simulink model "DC_DC_source_based_matrix_switches1_2022a"  (R2023a)
settings: Solver=FixedStepAuto  StartTime=0.0  StopTime=10000  RelTol=1e-3
InitFcn:
  | %run('D:\Thesis\main.m')
  | %run('E:\Thesis\main.m')
values from neighbouring files (symbols this model uses):
  cell_cap_Ah = 2.2    [find_maximum_ovlp.m]    (also in main.m)
  dst_q_cls = zeros(50, 2)    [main.m]
  dst_trg_soc_av = zeros(50, 1)    [main.m]
  soc = soc_in    [balance_costF.m]    (also in find_maximum_ovlp.m = fix(rand (1, cell_count) * 100); log_clustering.m; main.m = fix(rand (1, cell_count) * 100); plot_final.m)
  src_q_cls = zeros(50, 2)    [main.m]
  src_trg_soc_av = zeros(50, 1)    [main.m]
undefined symbols (not defined in the file or in its folder): Ion, Lithium
libraries: spsIdealSwitchLib x18, spsBatteryLib x9, spsControlledCurrentSourceLib x2, spsVoltageMeasurementLib x2, spsOnDelayLib x1, spsSeriesRLCBranchLib x1, spspowerguiLib x1
settings Model: Creator=Mahdi  LastModifiedBy=10661025
settings OptimizationCC: DefaultParameterBehavior=Inlined  EnhancedBackFolding=on  PassReuseOutputArgsAs=Individual arguments  ZeroExternalMemoryAtStartup=off  ZeroInternalMemoryAtStartup=off  OptimizeBlockOrder=speed  DifferentSizesBufferReuse=on  OptimizationCustomize=off  EfficientTunableParamExpr=on
settings DebuggingCC: ParameterTunabilityLossMsg=error
settings HardwareCC: ProdBitPerInt=16  ProdBitPerPointer=16  ProdBitPerSizeT=16  ProdBitPerPtrDiffT=16  ProdLargestAtomicFloat=None  ProdWordSize=16  ProdHWDeviceType=STMicroelectronics->ST10/Super10
settings ModelReferenceCC: ModelReferenceMinAlgLoopOccurrences=on
settings SFSimCC: MATLABDynamicMemAlloc=off
settings RTWCC: Description=Embedded Coder  SystemTargetFile=ert.tlc  TemplateMakefile=ert_default_tmf
settings CodeAppCC: ForceParamTrailComments=on  IgnoreCustomStorageClasses=off  OperatorAnnotations=on  SimulinkDataObjDesc=on  SFDataObjDesc=on  InsertBlockDesc=on
settings ERTTargetCC: TargetLangStandard=C99 (ISO)  GenerateSampleERTMain=on  SupportContinuousTime=on  SupportVariableSizeSignals=on  InlinedParameterPlacement=NonHierarchical  ERTCustomFileTemplate=example_file_process.tlc

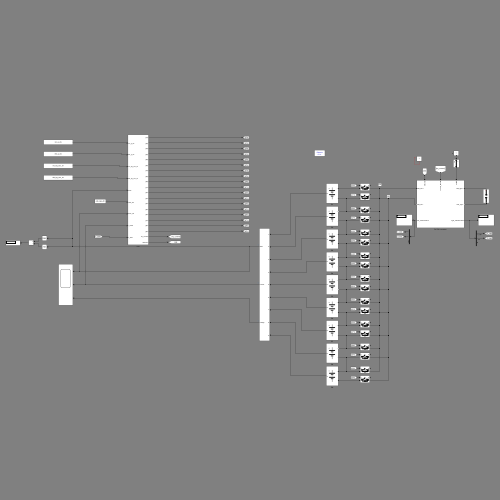
[thumbnail: Simulink's stored preview of the top-level diagram]
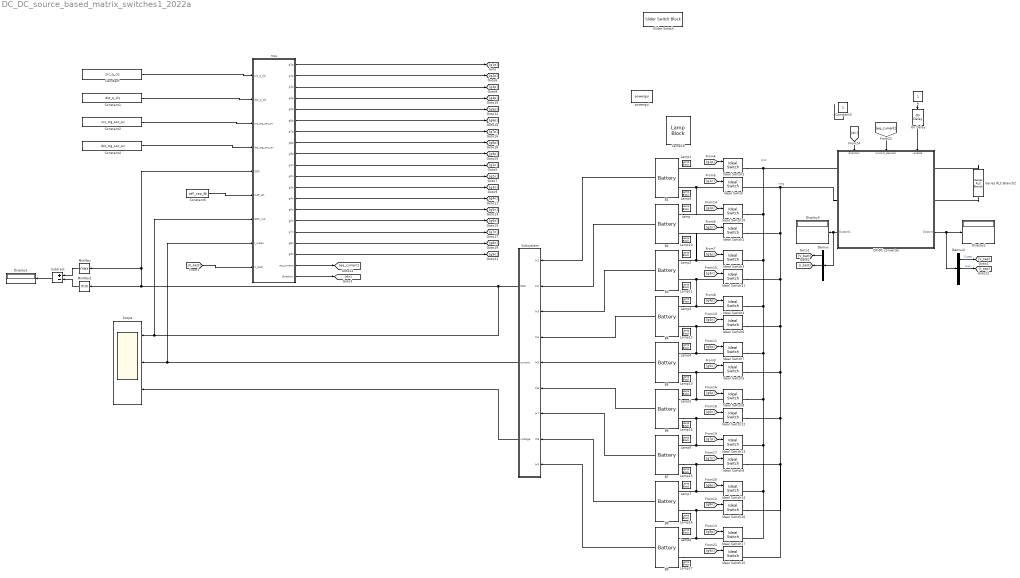
== system DC_DC_source_based_matrix_switches1_2022a ==
  note: pos
  note: neg
  B1 : spsBatteryLib/Battery  BatType=Lithium-Ion  ShowTempParam=off  ThermalPreset=no  ShowAgeParam=off  NomV=3.7  NomQ=2.2  SOC=soc(1, 1)  Batt_Tr=30  PresetModel=on  MaxQ=2.2  MinV=2.775  FullV=4.3068  Dis_rate=0.95652  R=0.016818  Normal_OP=1.9896  expZone="[3.9974     0.10809]"  current=[6.5 13 32.5]  Units=Time  Tci=20  NomT=20  T2=-30  MaxQ2=4.8  FullV2=7.1  Normal_OP2=5.655  expZone2="[6.58           1]"  Rca=0.6  ti=2000  Dp=0  Neq0=0  Tsim=1e6  Ta1=25  Qeol=5.4*0.9  Reol=0.013333*1.2  Char_age=[2.3478, 3]  Dis_age=[2.3478, 10]  N1=1500  N2=10500  N3=1000  N4=1400  Ta2=45  N5=950
  B2 : spsBatteryLib/Battery  BatType=Lithium-Ion  ShowTempParam=off  ThermalPreset=no  ShowAgeParam=off  NomV=3.7  NomQ=2.2  SOC=soc(1, 2)  Batt_Tr=30  PresetModel=on  MaxQ=2.2  MinV=2.775  FullV=4.3068  Dis_rate=0.95652  R=0.016818  Normal_OP=1.9896  expZone="[3.9974     0.10809]"  current=[6.5 13 32.5]  Units=Time  Tci=20  NomT=20  T2=-30  MaxQ2=4.8  FullV2=7.1  Normal_OP2=5.655  expZone2="[6.58           1]"  Rca=0.6  ti=2000  Dp=0  Neq0=0  Tsim=1e6  Ta1=25  Qeol=5.4*0.9  Reol=0.013333*1.2  Char_age=[2.3478, 3]  Dis_age=[2.3478, 10]  N1=1500  N2=10500  N3=1000  N4=1400  Ta2=45  N5=950
  B3 : spsBatteryLib/Battery  BatType=Lithium-Ion  ShowTempParam=off  ThermalPreset=no  ShowAgeParam=off  NomV=3.7  NomQ=2.2  SOC=soc(1, 3)  Batt_Tr=30  PresetModel=on  MaxQ=2.2  MinV=2.775  FullV=4.3068  Dis_rate=0.95652  R=0.016818  Normal_OP=1.9896  expZone="[3.9974     0.10809]"  current=[6.5 13 32.5]  Units=Time  Tci=20  NomT=20  T2=-30  MaxQ2=4.8  FullV2=7.1  Normal_OP2=5.655  expZone2="[6.58           1]"  Rca=0.6  ti=2000  Dp=0  Neq0=0  Tsim=1e6  Ta1=25  Qeol=5.4*0.9  Reol=0.013333*1.2  Char_age=[2.3478, 3]  Dis_age=[2.3478, 10]  N1=1500  N2=10500  N3=1000  N4=1400  Ta2=45  N5=950
  B4 : spsBatteryLib/Battery  BatType=Lithium-Ion  ShowTempParam=off  ThermalPreset=no  ShowAgeParam=off  NomV=3.7  NomQ=2.2  SOC=soc(1, 4)  Batt_Tr=30  PresetModel=on  MaxQ=2.2  MinV=2.775  FullV=4.3068  Dis_rate=0.95652  R=0.016818  Normal_OP=1.9896  expZone="[3.9974     0.10809]"  current=[6.5 13 32.5]  Units=Time  Tci=20  NomT=20  T2=-30  MaxQ2=4.8  FullV2=7.1  Normal_OP2=5.655  expZone2="[6.58           1]"  Rca=0.6  ti=2000  Dp=0  Neq0=0  Tsim=1e6  Ta1=25  Qeol=5.4*0.9  Reol=0.013333*1.2  Char_age=[2.3478, 3]  Dis_age=[2.3478, 10]  N1=1500  N2=10500  N3=1000  N4=1400  Ta2=45  N5=950
  B5 : spsBatteryLib/Battery  BatType=Lithium-Ion  ShowTempParam=off  ThermalPreset=no  ShowAgeParam=off  NomV=3.7  NomQ=2.2  SOC=soc(1, 5)  Batt_Tr=30  PresetModel=on  MaxQ=2.2  MinV=2.775  FullV=4.3068  Dis_rate=0.95652  R=0.016818  Normal_OP=1.9896  expZone="[3.9974     0.10809]"  current=[6.5 13 32.5]  Units=Time  Tci=20  NomT=20  T2=-30  MaxQ2=4.8  FullV2=7.1  Normal_OP2=5.655  expZone2="[6.58           1]"  Rca=0.6  ti=2000  Dp=0  Neq0=0  Tsim=1e6  Ta1=25  Qeol=5.4*0.9  Reol=0.013333*1.2  Char_age=[2.3478, 3]  Dis_age=[2.3478, 10]  N1=1500  N2=10500  N3=1000  N4=1400  Ta2=45  N5=950
  B6 : spsBatteryLib/Battery  BatType=Lithium-Ion  ShowTempParam=off  ThermalPreset=no  ShowAgeParam=off  NomV=3.7  NomQ=2.2  SOC=soc(1, 6)  Batt_Tr=30  PresetModel=on  MaxQ=2.2  MinV=2.775  FullV=4.3068  Dis_rate=0.95652  R=0.016818  Normal_OP=1.9896  expZone="[3.9974     0.10809]"  current=[6.5 13 32.5]  Units=Time  Tci=20  NomT=20  T2=-30  MaxQ2=4.8  FullV2=7.1  Normal_OP2=5.655  expZone2="[6.58           1]"  Rca=0.6  ti=2000  Dp=0  Neq0=0  Tsim=1e6  Ta1=25  Qeol=5.4*0.9  Reol=0.013333*1.2  Char_age=[2.3478, 3]  Dis_age=[2.3478, 10]  N1=1500  N2=10500  N3=1000  N4=1400  Ta2=45  N5=950
  B7 : spsBatteryLib/Battery  BatType=Lithium-Ion  ShowTempParam=off  ThermalPreset=no  ShowAgeParam=off  NomV=3.7  NomQ=2.2  SOC=soc(1, 7)  Batt_Tr=30  PresetModel=on  MaxQ=2.2  MinV=2.775  FullV=4.3068  Dis_rate=0.95652  R=0.016818  Normal_OP=1.9896  expZone="[3.9974     0.10809]"  current=[6.5 13 32.5]  Units=Time  Tci=20  NomT=20  T2=-30  MaxQ2=4.8  FullV2=7.1  Normal_OP2=5.655  expZone2="[6.58           1]"  Rca=0.6  ti=2000  Dp=0  Neq0=0  Tsim=1e6  Ta1=25  Qeol=5.4*0.9  Reol=0.013333*1.2  Char_age=[2.3478, 3]  Dis_age=[2.3478, 10]  N1=1500  N2=10500  N3=1000  N4=1400  Ta2=45  N5=950
  B8 : spsBatteryLib/Battery  BatType=Lithium-Ion  ShowTempParam=off  ThermalPreset=no  ShowAgeParam=off  NomV=3.7  NomQ=2.2  SOC=soc(1, 8)  Batt_Tr=30  PresetModel=on  MaxQ=2.2  MinV=2.775  FullV=4.3068  Dis_rate=0.95652  R=0.016818  Normal_OP=1.9896  expZone="[3.9974     0.10809]"  current=[6.5 13 32.5]  Units=Time  Tci=20  NomT=20  T2=-30  MaxQ2=4.8  FullV2=7.1  Normal_OP2=5.655  expZone2="[6.58           1]"  Rca=0.6  ti=2000  Dp=0  Neq0=0  Tsim=1e6  Ta1=25  Qeol=5.4*0.9  Reol=0.013333*1.2  Char_age=[2.3478, 3]  Dis_age=[2.3478, 10]  N1=1500  N2=10500  N3=1000  N4=1400  Ta2=45  N5=950
  B9 : spsBatteryLib/Battery  BatType=Lithium-Ion  ShowTempParam=off  ThermalPreset=no  ShowAgeParam=off  NomV=3.7  NomQ=2.2  SOC=soc(1, 9)  Batt_Tr=30  PresetModel=on  MaxQ=2.2  MinV=2.775  FullV=4.3068  Dis_rate=0.95652  R=0.016818  Normal_OP=1.9896  expZone="[3.9974     0.10809]"  current=[6.5 13 32.5]  Units=Time  Tci=20  NomT=20  T2=-30  MaxQ2=4.8  FullV2=7.1  Normal_OP2=5.655  expZone2="[6.58           1]"  Rca=0.6  ti=2000  Dp=0  Neq0=0  Tsim=1e6  Ta1=25  Qeol=5.4*0.9  Reol=0.013333*1.2  Char_age=[2.3478, 3]  Dis_age=[2.3478, 10]  N1=1500  N2=10500  N3=1000  N4=1400  Ta2=45  N5=950
  Constant : Constant  Value=src_q_cls
  Constant1 : Constant  Value=dst_q_cls
  Constant2 : Constant  Value=src_trg_soc_av
  Constant3 : Constant
  Constant4 : Constant  Value=dst_trg_soc_av
  Constant5 : Constant  Value=cell_cap_Ah
  DC-DC converter : Subsystem
      settings: PortSchema="{\"entries\":[{\"content\":{\"sides\":[{\"content\":{\"connectorIds\":[\"LConn1\",\"LConn2\",\"Out2\"]},\"type\":\"ConnectorPlacement.EquallySpacedRectSide\",\"uuid\":\"b8e9ea21-fc6f-4abe-9815-7c96c8754cc1\"},{\"content\":{\"connectorIds\":[\"RConn1\",\"RConn2\",\"Out1\"],\"side\":\"RIGHT\"},\"type\":\"ConnectorPlacement.EquallySpacedRectSide\",\"uuid\":\"546bb611-6f28-45af-a15a-a960a3093258\"},{\"content\":{\"connectorIds\":[\"In1\",\"In2\",\"In3\"],\"side\":\"TOP\"},\"type\":\"ConnectorPlacement.EquallySpacedRectSide\",\"uuid\":\"f1a81754-76ae-41da-bcef-17d54c1fc977\"}]},\"type\":\"ConnectorPlacement.EquallySpacedConnector\",\"uuid\":\"f395fac5-4dd1-431a-bb8e-7682cfb9cc98\"}],\"packageUris\":[\"http://schema.mathworks.com/mf0/Connector/R2020b\"],\"version\":\"1.0\"}"
  Demux : Demux  Outputs=3
  Demux2 : Demux  Outputs=3
  Display1 : Display
  Display2 : Display
  Display3 : Display
  Ideal Switch{,1..17} (18 alike) : spsIdealSwitchLib/Ideal Switch  Ron=0.001  Lon=0  IC=0  Rs=1e5  Cs=inf  Measurements=on
  Lamp{,1..18} (19 alike) : LampBlock  LabelPosition=Hide
  MinMax : MinMax  Function=max
  MinMax1 : MinMax
  On Delay : spsOnDelayLib/On Delay  DelayType=On delay  delay=1  ic=0  Ts=0
  Scope : Scope  NumInputPorts=3
  Series RLC Branch2 : spsSeriesRLCBranchLib/Series RLC Branch  LConnTagsString=__new0  RConnTagsString=__new0  BranchType=C  Resistance=1  Inductance=1e-3  SetiL0=off  InitialCurrent=0  Capacitance=500  Setx0=on  InitialVoltage=0  Measurements=Branch voltage and current
  Slider Switch : SliderSwitchBlock
      settings: Values={{'Off', 'On'}, [0 1]}
  Subsystem : Subsystem
  Subtract : Sum  Inputs=+-
  e : Constant
  mcu : Subsystem
  powergui : spspowerguiLib/powergui  Priority=1  SimulationMode=Discrete  SampleTime=0.1  frequency=60  Iterations=50  frequencyindice=0  Pbase=100e6  ErrMax=1e-4  UnitsV=kV  UnitsW=MW  buscounter=0  FunctionMessages=off  echomessages=off  EnableUseOfTLC=off  CurrentSourceSwitches=off  DisableSnubberDevices=off  DisableRonSwitches=off  DisableVfSwitches=off  DisplayEquations=off  AutomaticDiscreteSolvers=off  SolverType=Tustin/Backward Euler (TBE)  Interpol=off  ExternalGateDelay=off  methode=on  Ts=1000  x0status=blocks  SPID=off  SwTol=0  HookPort=off  NonlinearTolerance=1e-4  nMaxIteration=10  ContinueOnMaxIteration=off  RestoreLinks=warning  ResistiveCurrentMeasurement=off  Frange=[0:2:500]  Ylog=off  Xlog=on  ShowGrid=off  save=off  variable=ZData  structure=0  ZoomFFT=off  StartTime=0.0  cycles=1  DisplayStyle=1  fundamental=60  FreqAxis=off  MaxFrequency=1000  frequencyindicesteady=1  RmsSteady=1  display=off
  wires:
  e/1 -> On Delay/1
  [dir] -> DC-DC converter/1(direction)
  DC-DC converter/1(Outport) -> Display2/1, Demux2/1
  DC-DC converter/2(Outport1) -> Demux/1, Display3/1
  Demux2/1 -> [V_cap]  "V_cap"
  [g1p] -> Ideal Switch1/1
  [g1n] -> Ideal Switch/1
  [g2p] -> Ideal Switch10/1
  [g2n] -> Ideal Switch2/1
  [g3p] -> Ideal Switch3/1
  [g3n] -> Ideal Switch11/1
  [g5n] -> Ideal Switch5/1
  [g5p] -> Ideal Switch7/1
  [g4n] -> Ideal Switch6/1
  [g4p] -> Ideal Switch4/1
  [g8p] -> Ideal Switch14/1
  [g8n] -> Ideal Switch16/1
  [g9p] -> Ideal Switch17/1
  [g9n] -> Ideal Switch15/1
  [g7n] -> Ideal Switch9/1
  [g7p] -> Ideal Switch13/1
  [g6n] -> Ideal Switch12/1
  [g6p] -> Ideal Switch8/1
  [eq_current] -> DC-DC converter/2(current_desired)
  Demux/1 -> [V_batt]
  Demux/2 -> [I_batt]
  Demux2/2 -> [I_cap]  "Iout"
  Constant3/1 -> ?
  B1/1 -> Subsystem/1(In1)
  B2/1 -> Subsystem/2(In2)
  B3/1 -> Subsystem/3(In3)
  B4/1 -> Subsystem/4(In4)
  B5/1 -> Subsystem/5(In5)
  B6/1 -> Subsystem/6(In6)
  B7/1 -> Subsystem/7(In7)
  B8/1 -> Subsystem/8(In8)
  B9/1 -> Subsystem/9(In9)
  Subsystem/2(current) -> mcu/8(I_meas), Scope/2
  Subsystem/3(voltage) -> Scope/3
  MinMax/1 -> Subtract/1
  MinMax1/1 -> Subtract/2
  Subtract/1 -> Display1/1
  Constant/1 -> mcu/1(src_q_cls)
  Constant1/1 -> mcu/2(dst_q_cls)
  Constant2/1 -> mcu/3(src_trg_soc_av)
  Constant4/1 -> mcu/4(dst_trg_soc_av)
  mcu/1(g1p) -> [g1p]
  mcu/2(g2p) -> [g2p]
  mcu/3(g3p) -> [g3p]
  mcu/4(g4p) -> [g4p]
  mcu/5(g5p) -> [g5p]
  mcu/6(g6p) -> [g6p]
  mcu/7(g7p) -> [g7p]
  mcu/8(g8p) -> [g8p]
  mcu/9(g9p) -> [g9p]
  mcu/10(g1n) -> [g1n]
  mcu/11(g2n) -> [g2n]
  mcu/12(g3n) -> [g3n]
  mcu/13(g4n) -> [g4n]
  mcu/14(g5n) -> [g5n]
  mcu/15(g6n) -> [g6n]
  mcu/16(g7n) -> [g7n]
  mcu/17(g8n) -> [g8n]
  mcu/18(g9n) -> [g9n]
  Constant5/1 -> mcu/6(CAP_Ah)
  Subsystem/1(SOC) -> MinMax/1, mcu/5(SOC), MinMax1/1, Scope/1, mcu/7(SOC_init)
  mcu/19(eq_current) -> [eq_current]
  [V_batt] -> mcu/9(V_batt)
  mcu/20(direction) -> [dir]
  On Delay/1 -> DC-DC converter/3(enable)
  connections:
  Series RLC Branch2/LConn1 -- DC-DC converter/RConn1
  Series RLC Branch2/RConn1 -- DC-DC converter/RConn2
  Ideal Switch/LConn1 -- Ideal Switch10/LConn1 -- B2/LConn1 -- B1/LConn2
  Ideal Switch1/LConn1 -- B1/LConn1
  Ideal Switch2/LConn1 -- B2/LConn2 -- Ideal Switch3/LConn1 -- B3/LConn1
  B4/LConn1 -- Ideal Switch11/LConn1 -- B3/LConn2 -- Ideal Switch4/LConn1
  B4/LConn2 -- Ideal Switch6/LConn1 -- Ideal Switch7/LConn1 -- B5/LConn1
  B6/LConn1 -- Ideal Switch5/LConn1 -- B5/LConn2 -- Ideal Switch8/LConn1
  B6/LConn2 -- Ideal Switch12/LConn1 -- Ideal Switch13/LConn1 -- B7/LConn1
  B7/LConn2 -- Ideal Switch9/LConn1 -- B8/LConn1 -- Ideal Switch14/LConn1
  B8/LConn2 -- Ideal Switch17/LConn1 -- B9/LConn1 -- Ideal Switch16/LConn1
  Ideal Switch16/RConn1 -- Ideal Switch15/RConn1 -- Ideal Switch9/RConn1 -- Ideal Switch12/RConn1 -- Ideal Switch5/RConn1 -- Ideal Switch6/RConn1 -- Ideal Switch11/RConn1 -- Ideal Switch2/RConn1 -- DC-DC converter/LConn2 -- Ideal Switch/RConn1
  Ideal Switch1/RConn1 -- DC-DC converter/LConn1 -- Ideal Switch10/RConn1 -- Ideal Switch3/RConn1 -- Ideal Switch4/RConn1 -- Ideal Switch7/RConn1 -- Ideal Switch17/RConn1 -- Ideal Switch14/RConn1 -- Ideal Switch13/RConn1 -- Ideal Switch8/RConn1
  B9/LConn2 -- Ideal Switch15/LConn1

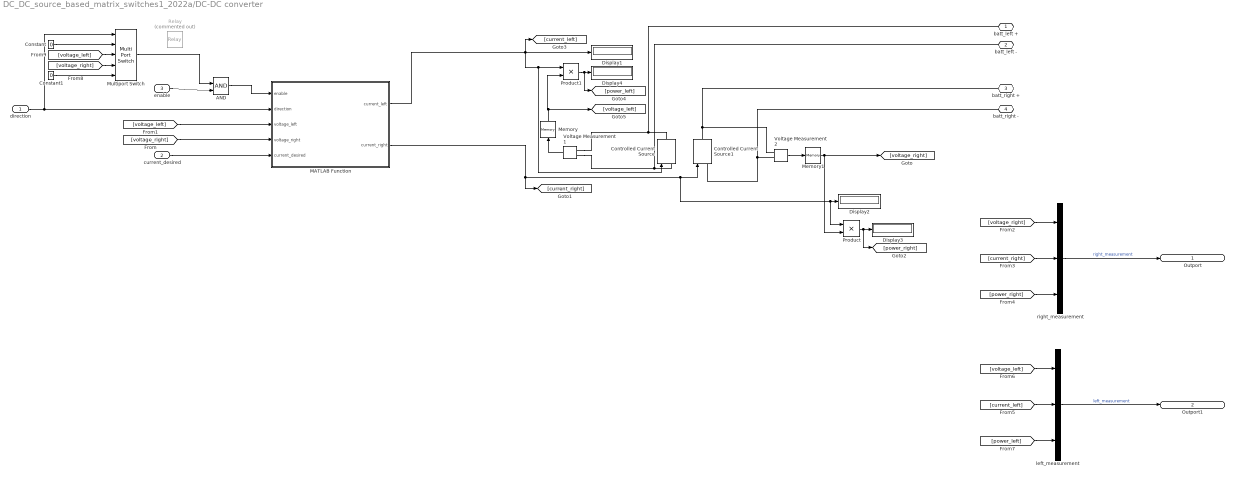
== system DC_DC_source_based_matrix_switches1_2022a/DC-DC converter ==
  direction : Inport
  current_desired : Inport  Port=2
  enable : Inport  Port=3
  AND : Logic  IconShape=distinctive  AllPortsSameDT=off  OutDataTypeStr=boolean
  Constant : Constant  Value=0
  Constant1 : Constant  Value=0
  Controlled Current Source : spsControlledCurrentSourceLib/Controlled Current Source  Initialize=on  Source_Type=DC  Amplitude=0  Phase=0  Frequency=0  Measurements=None
  Controlled Current Source1 : spsControlledCurrentSourceLib/Controlled Current Source  Initialize=on  Source_Type=AC  Amplitude=0  Phase=0  Frequency=0  Measurements=None
  Display{1..4} (4 alike) : Display
  MATLAB Function : MATLAB Function  TreatAsAtomicUnit=on
  Memory : Memory
  Memory1 : Memory
  Multiport Switch : MultiPortSwitch  DataPortOrder=Zero-based contiguous  DataPortForDefault=Additional data port  zeroidx=on  SaturateOnIntegerOverflow=off  InputSameDT=off
  Product : Product
  Product1 : Product
  Relay : Relay  Commented=on  OnSwitchValue=3.5  OffSwitchValue=2
  Voltage Measurement1 : spsVoltageMeasurementLib/Voltage Measurement  PhasorSimulation=off  OutputType=Complex  PSBequivalent=0
  Voltage Measurement2 : spsVoltageMeasurementLib/Voltage Measurement  PhasorSimulation=off  OutputType=Complex  PSBequivalent=0
  left_measurement : Mux  Inputs=3
  right_measurement : Mux  Inputs=3
  batt_left + : PMIOPort  Side=Left
  batt_left - : PMIOPort  Port=2  Side=Left
  batt_right + : PMIOPort  Port=3  Side=Right
  batt_right - : PMIOPort  Port=4  Side=Right
  Outport : Outport
  Outport1 : Outport  Port=2
  wires:
  MATLAB Function/1(current_left) -> Controlled Current Source/1, Product1/1, [current_left], Display1/1
  enable/1 -> AND/2
  Voltage Measurement2/1 -> Memory1/1
  direction/1 -> MATLAB Function/2(direction), Multiport Switch/1
  [voltage_right] -> MATLAB Function/4(voltage_right)
  MATLAB Function/2(current_right) -> [current_right], Product/1, Display2/1, Controlled Current Source1/1
  [voltage_left] -> MATLAB Function/3(voltage_left)
  Product/1 -> [power_right], Display3/1
  Product1/1 -> [power_left], Display4/1
  current_desired/1 -> MATLAB Function/5(current_desired)
  [voltage_right] -> right_measurement/1
  [current_right] -> right_measurement/2
  [power_right] -> right_measurement/3
  [power_left] -> left_measurement/3
  [current_left] -> left_measurement/2
  [voltage_left] -> left_measurement/1
  right_measurement/1 -> Outport/1  "right_measurement"
  left_measurement/1 -> Outport1/1  "left_measurement"
  Voltage Measurement1/1 -> Memory/1
  Multiport Switch/1 -> AND/1
  AND/1 -> MATLAB Function/1(enable)
  Memory/1 -> Product1/2, [voltage_left]
  Memory1/1 -> [voltage_right], Product/2
  [voltage_left] -> Multiport Switch/3
  [voltage_right] -> Multiport Switch/4
  Constant/1 -> Multiport Switch/2
  Constant1/1 -> Multiport Switch/5
  connections:
  Voltage Measurement1/LConn1 -- batt_left +/RConn1 -- Controlled Current Source/RConn1
  Controlled Current Source1/RConn1 -- batt_right +/RConn1 -- Voltage Measurement2/LConn1
  Voltage Measurement2/LConn2 -- Controlled Current Source1/LConn1 -- batt_right -/RConn1
  Voltage Measurement1/LConn2 -- batt_left -/RConn1 -- Controlled Current Source/LConn1

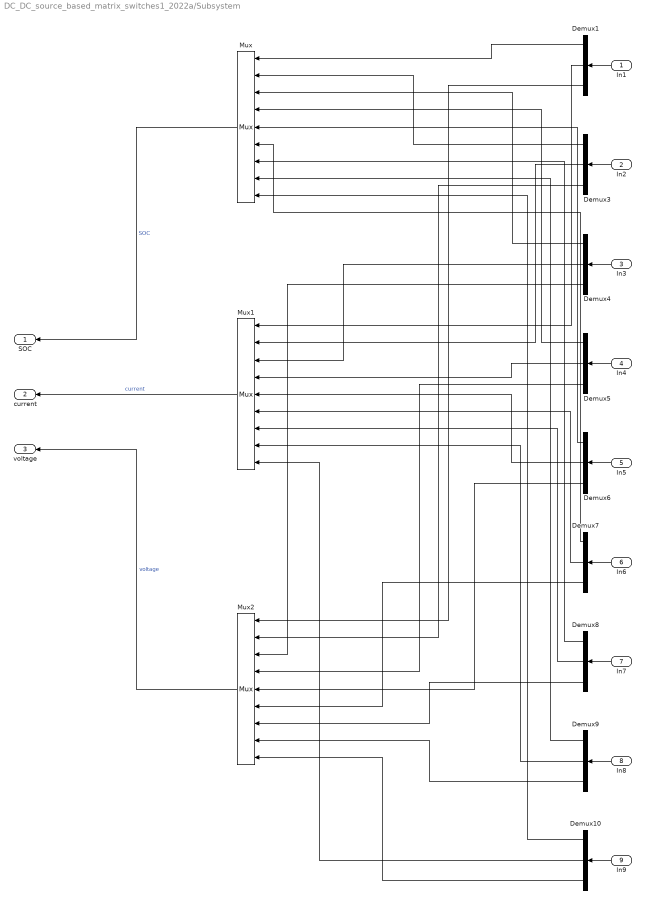
== system DC_DC_source_based_matrix_switches1_2022a/Subsystem ==
  In1 : Inport
  In2 : Inport  Port=2
  In3 : Inport  Port=3
  In4 : Inport  Port=4
  In5 : Inport  Port=5
  In6 : Inport  Port=6
  In7 : Inport  Port=7
  In8 : Inport  Port=8
  In9 : Inport  Port=9
  Demux{1,3..10} (9 alike) : Demux  Outputs=3
  Mux : Mux  Inputs=9
  Mux1 : Mux  Inputs=9
  Mux2 : Mux  Inputs=9
  SOC : Outport
  current : Outport  Port=2
  voltage : Outport  Port=3
  wires:
  In7/1 -> Demux8/1
  Demux6/3 -> Mux2/5
  Demux8/3 -> Mux2/7
  In5/1 -> Demux6/1
  Demux7/3 -> Mux2/6
  Demux4/1 -> Mux/3
  Demux10/3 -> Mux2/9
  Mux1/1 -> current/1  "current"
  Demux4/2 -> Mux1/3
  Demux1/3 -> Mux2/1
  Demux5/3 -> Mux2/4
  Demux10/1 -> Mux/9
  Demux4/3 -> Mux2/3
  Demux9/2 -> Mux1/8
  Demux9/3 -> Mux2/8
  Demux3/3 -> Mux2/2
  Demux9/1 -> Mux/8
  Demux10/2 -> Mux1/9
  Demux8/2 -> Mux1/7
  Demux3/1 -> Mux/2
  In6/1 -> Demux7/1
  Demux1/2 -> Mux1/1
  Demux6/1 -> Mux/5
  Demux8/1 -> Mux/7
  In1/1 -> Demux1/1
  In9/1 -> Demux10/1
  Demux7/1 -> Mux/6
  Demux1/1 -> Mux/1
  Demux3/2 -> Mux1/2
  Demux5/1 -> Mux/4
  Demux5/2 -> Mux1/4
  Demux6/2 -> Mux1/5
  Demux7/2 -> Mux1/6
  Mux/1 -> SOC/1  "SOC"
  In2/1 -> Demux3/1
  Mux2/1 -> voltage/1  "voltage"
  In3/1 -> Demux4/1
  In4/1 -> Demux5/1
  In8/1 -> Demux9/1

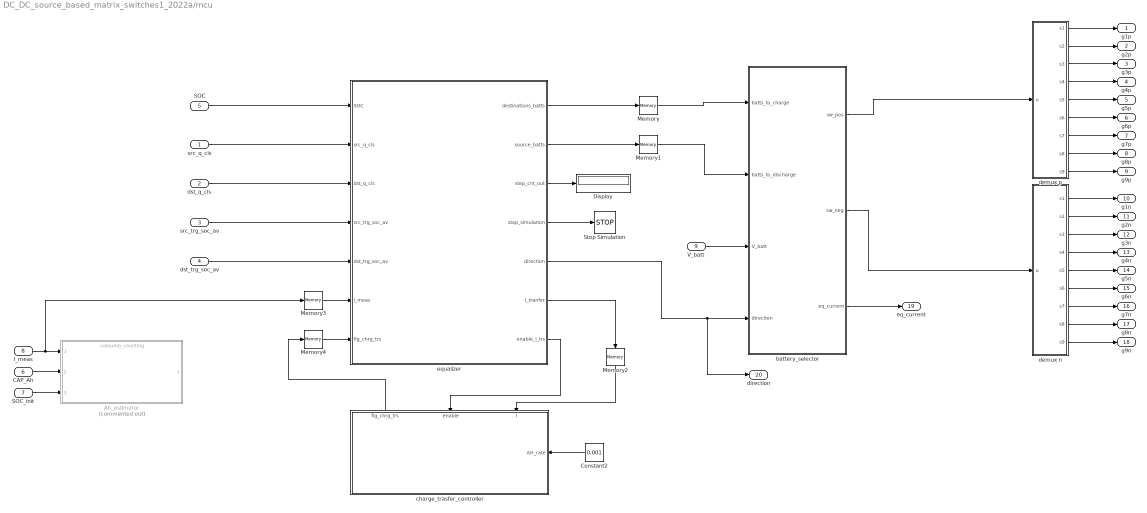
== system DC_DC_source_based_matrix_switches1_2022a/mcu ==
  src_q_cls : Inport
  dst_q_cls : Inport  Port=2
  src_trg_soc_av : Inport  Port=3
  dst_trg_soc_av : Inport  Port=4
  SOC : Inport  Port=5
  CAP_Ah : Inport  Port=6
  SOC_init : Inport  Port=7
  I_meas : Inport  Port=8
  V_batt : Inport  Port=9
  Ah_estimator : ModelReference  Commented=on  ModelNameDialog=coloumb_counting.slx  SimulationMode=Normal  ModelReferenceVersion=1.13
  Constant2 : Constant  Value=0.001
  Display : Display
  Memory{,1..4} (5 alike) : Memory
  Stop Simulation : Stop
  battery_selector : MATLAB Function  TreatAsAtomicUnit=on
  charge_trasfer_controller : Subsystem
      settings: PortSchema="{\"entries\":[{\"content\":{\"sides\":[{\"content\":{},\"type\":\"ConnectorPlacement.EquallySpacedRectSide\",\"uuid\":\"48c70ec0-4261-4909-a719-c03e97c3e4ca\"},{\"content\":{\"connectorIds\":[\"In3\"],\"side\":\"RIGHT\"},\"type\":\"ConnectorPlacement.EquallySpacedRectSide\",\"uuid\":\"8a44a88a-c632-4005-90b8-1b0d09211c10\"},{\"content\":{\"connectorIds\":[\"Out1\",\"In1\",\"In2\"],\"side\":\"TOP\"},\"type\":\"ConnectorPlacement.EquallySpacedRectSide\",\"uuid\":\"71bafe47-820a-4a08-9919-e54bf550fba8\"}]},\"type\":\"ConnectorPlacement.EquallySpacedConnector\",\"uuid\":\"9c996bd2-099e-4131-a64b-67fbb4a72a45\"}],\"packageUris\":[\"http://schema.mathworks.com/mf0/Connector/R2020b\"],\"version\":\"1.0\"}"
  demux n : MATLAB Function  TreatAsAtomicUnit=on
  demux p : MATLAB Function  TreatAsAtomicUnit=on
  equalizer : MATLAB Function  TreatAsAtomicUnit=on
  g1p : Outport
  g2p : Outport  Port=2
  g3p : Outport  Port=3
  g4p : Outport  Port=4
  g5p : Outport  Port=5
  g6p : Outport  Port=6
  g7p : Outport  Port=7
  g8p : Outport  Port=8
  g9p : Outport  Port=9
  g1n : Outport  Port=10
  g2n : Outport  Port=11
  g3n : Outport  Port=12
  g4n : Outport  Port=13
  g5n : Outport  Port=14
  g6n : Outport  Port=15
  g7n : Outport  Port=16
  g8n : Outport  Port=17
  g9n : Outport  Port=18
  eq_current : Outport  Port=19
  direction : Outport  Port=20
  wires:
  battery_selector/3(eq_current) -> eq_current/1
  Memory/1 -> battery_selector/1(batts_to_charge)
  demux n/3(s3) -> g3n/1
  demux n/7(s7) -> g7n/1
  demux n/2(s2) -> g2n/1
  equalizer/1(destinations_batts) -> Memory/1
  dst_q_cls/1 -> equalizer/3(dst_q_cls)
  equalizer/4(stop_simulation) -> Stop Simulation/1
  demux p/7(s7) -> g7p/1
  Memory1/1 -> battery_selector/2(batts_to_discharge)
  demux n/6(s6) -> g6n/1
  battery_selector/1(sw_pos) -> demux p/1(u)
  equalizer/2(source_batts) -> Memory1/1
  equalizer/3(step_cnt_out) -> Display/1
  battery_selector/2(sw_neg) -> demux n/1(u)
  src_q_cls/1 -> equalizer/2(src_q_cls)
  src_trg_soc_av/1 -> equalizer/4(src_trg_soc_av)
  demux n/5(s5) -> g5n/1
  demux n/8(s8) -> g8n/1
  dst_trg_soc_av/1 -> equalizer/5(dst_trg_soc_av)
  demux p/9(s9) -> g9p/1
  demux p/4(s4) -> g4p/1
  demux p/1(s1) -> g1p/1
  SOC/1 -> equalizer/1(SOC)
  demux p/5(s5) -> g5p/1
  demux p/2(s2) -> g2p/1
  demux p/8(s8) -> g8p/1
  demux n/1(s1) -> g1n/1
  demux n/4(s4) -> g4n/1
  demux n/9(s9) -> g9n/1
  demux p/3(s3) -> g3p/1
  demux p/6(s6) -> g6p/1
  SOC_init/1 -> Ah_estimator/3
  CAP_Ah/1 -> Ah_estimator/2
  Constant2/1 -> charge_trasfer_controller/3(AH_rate)
  equalizer/6(I_tranfer) -> Memory2/1
  equalizer/7(enable_I_trs) -> charge_trasfer_controller/1(enable)
  charge_trasfer_controller/1(flg_chrg_trs) -> Memory4/1
  equalizer/5(direction) -> direction/1, battery_selector/4(direction)
  I_meas/1 -> Memory3/1, Ah_estimator/1
  Memory2/1 -> charge_trasfer_controller/2(I)
  Memory3/1 -> equalizer/6(I_meas)
  Memory4/1 -> equalizer/7(flg_chrg_trs)
  V_batt/1 -> battery_selector/3(V_batt)

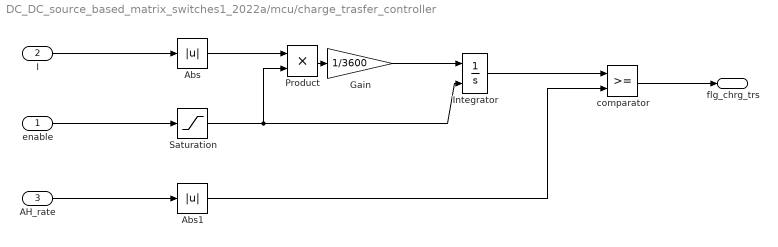
== system DC_DC_source_based_matrix_switches1_2022a/mcu/charge_trasfer_controller ==
  enable : Inport
  I : Inport  Port=2
  AH_rate : Inport  Port=3
  Abs : Abs  SaturateOnIntegerOverflow=off
  Abs1 : Abs  SaturateOnIntegerOverflow=off
  Gain : Gain  Gain=1/3600
  Integrator : Integrator  ExternalReset=either
  Product : Product
  Saturation : Saturate  UpperLimit=1  LowerLimit=0
  comparator : RelationalOperator  OutDataTypeStr=boolean  RndMeth=Simplest  InputSameDT=off
  flg_chrg_trs : Outport
  wires:
  comparator/1 -> flg_chrg_trs/1
  AH_rate/1 -> Abs1/1
  Abs/1 -> Product/1
  Integrator/1 -> comparator/1
  Product/1 -> Gain/1
  enable/1 -> Saturation/1
  Gain/1 -> Integrator/1
  Saturation/1 -> Product/2, Integrator/2
  I/1 -> Abs/1
  Abs1/1 -> comparator/2

== matlab function DC_DC_source_based_matrix_switches1_2022a/mcu/battery_selector ==
  data: batts_to_charge input; sw_pos output; sw_neg output; batts_to_discharge input; V_batt input; direction input; eq_current output
function [sw_pos, sw_neg, eq_current] = battery_selector(batts_to_charge, batts_to_discharge, V_batt, direction)
    persistent direction_pre;
    sw_pos = 0;
    sw_neg = 0;
    eq_current = 0;
    eq_current_tmp = 0;
    if isempty(direction_pre)
        direction_pre = 0;
    end
% to prevent invalid switch selection
if ( batts_to_charge(1, 1) <= batts_to_charge(1, 2) && ...
     batts_to_discharge(1, 1) <= batts_to_discharge(1, 2))
    
    % charge the capacitor using batteries
    if(direction == 1)
        if direction_pre ~= direction
            eq_current_tmp = 0;
            direction_pre = direction;
        else
            sw_pos = batts_to_discharge(1, 1);
            sw_neg = batts_to_discharge(1, 2);
            eq_current_tmp = 4;        
        end
    % charge the battery using capacitor
    elseif(direction == 2)
        if direction_pre ~= direction
            eq_current_tmp = 0;
            direction_pre = direction;
        else
            sw_pos = batts_to_charge(1, 1);
            sw_neg = batts_to_charge(1, 2);
            eq_current_tmp = 4;
        end
    else
        sw_pos = 0;
        sw_neg = 0;

    end

    if(V_batt < 2)
        eq_current = 0;
    else
        eq_current = eq_current_tmp * 0.5;
    end

end


end

== matlab function DC_DC_source_based_matrix_switches1_2022a/DC-DC converter/MATLAB Function ==
  data: enable input; current_left output; direction input; voltage_left input; voltage_right input; current_right output; current_desired input
function [current_left, current_right] = current_controller(enable, direction, voltage_left, voltage_right, current_desired)    
    current_left = 0;
    current_right = 0;
if(enable)
    %% left side sink, right side source
    if(direction == 1) 
        % variables definition
        current_sink = -1 * current_desired;
        voltage_sink = voltage_left;
        voltage_source = voltage_right;
        power_source = 0;
        power_sink = 0;

        % input and output power must match
        power_sink = current_sink * voltage_sink;
        power_source = power_sink;
        if(voltage_source ~= 0)
            current_source =  -1 * (power_source / voltage_source);
        else
            current_source = -1 * current_sink;
        end
        % power delivery
        if(current_sink > 0)
            current_sink = current_sink * -1;
        end
        if(current_source < 0)
            current_source = current_source * -1;
        end
        current_left = current_sink;
        current_right = current_source;
    %% right side source, left side sink
    elseif(direction == 2)
        % variables definition
        current_sink = -1 * current_desired;
        voltage_sink = voltage_right;
        voltage_source = voltage_left;
        power_source = 0;
        power_sink = 0;

        % input and output power must match
        power_sink = current_sink * voltage_sink;
        power_source = power_sink;
        if(voltage_source ~= 0)
            current_source =  -1 * (power_source / voltage_source);
        else
            current_source = -1 * current_sink;
        end
        % power delivery
        current_left = current_source;
        current_right = current_sink;
    end

else
    current_left = 0;
    current_right = 0;
end
end

== matlab function DC_DC_source_based_matrix_switches1_2022a/mcu/demux p ==
  data: u input; s1 output; s2 output; s3 output; s4 output; s5 output; s6 output; s7 output; s8 output; s9 output
function [s1, s2, s3, s4, s5, s6, s7, s8, s9] = demux(u)

    switch(u)
        case 1
            s1 = 1; s2 = 0;	s3 = 0; s4 = 0; s5 = 0; s6 = 0; s7 = 0; s8 = 0; s9 = 0;
        case 2      	
            s1 = 0; s2 = 1;	s3 = 0; s4 = 0; s5 = 0; s6 = 0; s7 = 0; s8 = 0; s9 = 0;
        case 3      	
            s1 = 0; s2 = 0;	s3 = 1; s4 = 0; s5 = 0; s6 = 0; s7 = 0; s8 = 0; s9 = 0;
        case 4      	
            s1 = 0; s2 = 0;	s3 = 0; s4 = 1; s5 = 0; s6 = 0; s7 = 0; s8 = 0; s9 = 0;
        case 5      	
            s1 = 0; s2 = 0;	s3 = 0; s4 = 0; s5 = 1; s6 = 0; s7 = 0; s8 = 0; s9 = 0;
        case 6      	
            s1 = 0; s2 = 0;	s3 = 0; s4 = 0; s5 = 0; s6 = 1; s7 = 0; s8 = 0; s9 = 0;
        case 7      
            s1 = 0; s2 = 0;	s3 = 0; s4 = 0; s5 = 0; s6 = 0; s7 = 1; s8 = 0; s9 = 0;
        case 8      	
            s1 = 0; s2 = 0;	s3 = 0; s4 = 0; s5 = 0; s6 = 0; s7 = 0; s8 = 1; s9 = 0;
        case 9      
            s1 = 0; s2 = 0;	s3 = 0; s4 = 0; s5 = 0; s6 = 0; s7 = 0; s8 = 0; s9 = 1;
        otherwise   	
            s1 = 0; s2 = 0;	s3 = 0; s4 = 0; s5 = 0; s6 = 0; s7 = 0; s8 = 0; s9 = 0;
    end
end

== matlab function DC_DC_source_based_matrix_switches1_2022a/mcu/demux n ==
  data: u input; s1 output; s2 output; s3 output; s4 output; s5 output; s6 output; s7 output; s8 output; s9 output
function [s1, s2, s3, s4, s5, s6, s7, s8, s9] = demux(u)

    switch(u)
        case 1
            s1 = 1; s2 = 0;	s3 = 0; s4 = 0; s5 = 0; s6 = 0; s7 = 0; s8 = 0; s9 = 0;
        case 2      	
            s1 = 0; s2 = 1;	s3 = 0; s4 = 0; s5 = 0; s6 = 0; s7 = 0; s8 = 0; s9 = 0;
        case 3      	
            s1 = 0; s2 = 0;	s3 = 1; s4 = 0; s5 = 0; s6 = 0; s7 = 0; s8 = 0; s9 = 0;
        case 4      	
            s1 = 0; s2 = 0;	s3 = 0; s4 = 1; s5 = 0; s6 = 0; s7 = 0; s8 = 0; s9 = 0;
        case 5      	
            s1 = 0; s2 = 0;	s3 = 0; s4 = 0; s5 = 1; s6 = 0; s7 = 0; s8 = 0; s9 = 0;
        case 6      	
            s1 = 0; s2 = 0;	s3 = 0; s4 = 0; s5 = 0; s6 = 1; s7 = 0; s8 = 0; s9 = 0;
        case 7      
            s1 = 0; s2 = 0;	s3 = 0; s4 = 0; s5 = 0; s6 = 0; s7 = 1; s8 = 0; s9 = 0;
        case 8      	
            s1 = 0; s2 = 0;	s3 = 0; s4 = 0; s5 = 0; s6 = 0; s7 = 0; s8 = 1; s9 = 0;
        case 9      
            s1 = 0; s2 = 0;	s3 = 0; s4 = 0; s5 = 0; s6 = 0; s7 = 0; s8 = 0; s9 = 1;
        otherwise   	
            s1 = 0; s2 = 0;	s3 = 0; s4 = 0; s5 = 0; s6 = 0; s7 = 0; s8 = 0; s9 = 0;
    end
end

== matlab function DC_DC_source_based_matrix_switches1_2022a/mcu/equalizer ==
  data: destinations_batts output; SOC input; source_batts output [..50]; src_q_cls input; dst_q_cls input; src_trg_soc_av input; dst_trg_soc_av input; I_meas input; step_cnt_out output; stop_simulation output; direction output; I_tranfer output; enable_I_trs output; flg_chrg_trs input
function [destinations_batts, source_batts, step_cnt_out, stop_simulation, direction, I_tranfer, enable_I_trs] = battery_selector(SOC, src_q_cls, dst_q_cls, src_trg_soc_av, dst_trg_soc_av, I_meas, flg_chrg_trs)


I_tranfer  = 0;
stop_simulation  = 0;
source_batts = [0 0];
destinations_batts = [0 0];
dst_trg_soc_av_tmp = dst_trg_soc_av;
src_trg_soc_av_tmp = src_trg_soc_av;

dst_trg_soc_av_tmp(dst_trg_soc_av == 0) = Inf;
% src_trg_soc_av_tmp(src_trg_soc_av == 0) = Inf;
% the number of steps to equlalize the battery pack
step = length(src_q_cls);

persistent step_cnt;
persistent I_cells_source;
persistent I_cells_destination;
persistent dir;
persistent enable;



if isempty(step_cnt)
    step_cnt = 1;
    assert(1, 'Simulation terminated because x >= 10')

end

if isempty(I_cells_source)
    I_cells_source = 0;
end
if isempty(I_cells_destination)
    I_cells_destination = 0;
end
if isempty(dir)
    dir = 0;
end
if isempty(enable)
    enable = 0;
end



soc = SOC';
if src_q_cls(step_cnt, :) > 0


    source_batts = src_q_cls(step_cnt, :);
    I_cells_source = I_meas(source_batts(1, 1));       % source cells current
    destinations_batts = dst_q_cls(step_cnt, :);
    I_cells_destination = I_meas(destinations_batts(1, 1));  % destication cells current



    if(dir == 0 && flg_chrg_trs == 0) % dischaege source if in the begining of charge transfering
        enable = 1; % start counting coulombs
        dir = 1; 
    end



    if(dir == 1 && flg_chrg_trs == 1 && enable == 1) % reset the flag
        enable = 0;
    end

    if(dir == 1 && flg_chrg_trs == 0 && enable == 0) % charge the destination if the prevoius charge transfer terminated
        enable = 1;
        dir = 2;
    end

    if(dir == 2 && flg_chrg_trs == 1 && enable == 1) % reset the flag
        enable = 0;
    end

    if(dir == 2 && flg_chrg_trs == 0 && enable == 0) % charge transfer terminated
        dir = 0;
    end

    if dir == 1
        I_tranfer = I_cells_source;
    elseif dir == 2
        I_tranfer = I_cells_destination;
    else
        I_tranfer = 0;
    end
    
    
    sm = mean(soc(src_q_cls(step_cnt, 1):src_q_cls(step_cnt, 2)));
    dm = mean(soc(dst_q_cls(step_cnt, 1):dst_q_cls(step_cnt, 2)));
    if(sm <= src_trg_soc_av_tmp(step_cnt) || dm >= dst_trg_soc_av_tmp(step_cnt)) && dir == 0
        step_cnt = step_cnt + 1;
    end
else
    direction = 0;
    I_cells_source = 0;
    I_cells_destination = 0;
    dir = 0;
    stop_simulation  = 1;
    enable = 0
end
direction = dir;
enable_I_trs = enable;


step_cnt_out = step_cnt;

end
